simulink library "pixhawk_slib_uORB_RW"  (R2017b)
settings: Solver=ode45  StartTime=0.0  StopTime=10.0  RelTol=1e-3
undefined symbols (not defined in the file or in its folder): UNDEFINED, uORB_StuctParams
settings Model: Creator=skuznick  LastModifiedBy=uavcs
settings DataIOCC: LimitDataPoints=on  SaveFormat=Array
settings OptimizationCC: BlockReduction=off  BooleanDataType=off  LifeSpan=inf
settings DebuggingCC: SaveWithParameterizedLinksMsg=none  UnderspecifiedInitializationDetection=Classic  MergeDetectMultiDrivingBlocksExec=none  SignalResolutionControl=TryResolveAllWithWarning  AllowSymbolicDim=off  StrictBusMsg=Warning  SFUnexpectedBacktrackingDiag=warning  SFNoUnconditionalDefaultTransitionDiag=warning  SFExecutionAtInitializationDiag=none
settings HardwareCC: ProdBitPerPointer=32  ProdBitPerSizeT=32  ProdBitPerPtrDiffT=32  ProdLargestAtomicFloat=None  ProdIntDivRoundTo=Undefined  ProdEndianess=Unspecified  ProdWordSize=32  ProdHWDeviceType=32-bit Generic  TargetUnknown=on
settings ModelReferenceCC: PropagateSignalLabelsOutOfModel=off
settings CodeAppCC: StateflowObjectComments=on
settings GRTTargetCC: TargetLangStandard=C89/C90 (ANSI)  GeneratePreprocessorConditionals=Disable all
settings ConfigComp: CovMetricSettings=dw  CovHtmlReporting=on  CovSaveCumulativeToWorkspaceVar=on  CovSaveSingleToWorkspaceVar=on  CovExternalEMLEnable=off  CovSFcnEnable=off

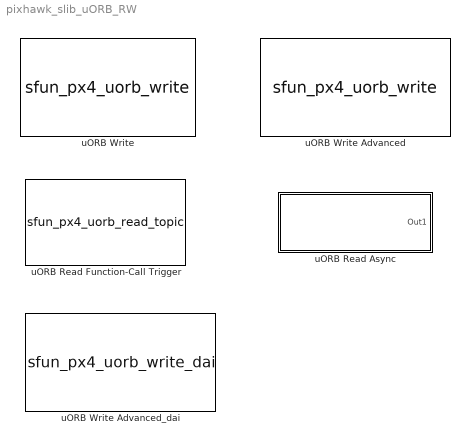
== system pixhawk_slib_uORB_RW ==
  uORB Read Async : Subsystem  mask{uORB_Topic_str=UNDEFINED, BusObjVar=Bus: actuator_armed_SL}
      mask prompts: BusObjVar "Enter Bus Object"
      mask help:
      | uORB Read Input Block
      |
      | Subscribes to a user provided named tropic structure.
      mask init:
      | ParentSubsystem = getSimulinkBlockHandle(get(gcbh,'parent'));
      | ParentConnection = [];
      | h_ParentSourceBlk = [];
      | err = 0;
      | if (ParentSubsystem~=-1)
      |     ParentConnection = get(ParentSubsystem,'PortConnectivity');
      | else
      |     set_param(gcb,'uORB_Topic_str','UNDEFINED');
      |     err = 1;
      | end
      | 
      | if ~isempty(ParentConnection)
      |     %Find which source block is the trigger
      |     for trigger_indx = 1:length(ParentConnection)
      |         if isequal(ParentConnection(trigger_indx).Type,'trigger')
      |             h_ParentSourceBlk = ParentConnection(trigger_indx).SrcBlock;
      |         end
      |     end
      | else
      |     set_param(gcb,'uORB_Topic_str','UNDEFINED');
      |     err = 1;
      | end
      | 
      | if ~isempty(h_ParentSourceBlk)
      | 
      |     Blk_Connections = get(h_ParentSourceBlk,'PortConnectivity');   
      | 
      |     while (1)
      |         Blk_Connections = get(h_ParentSourceBlk,'PortConnectivity');    
      |         if isempty(Blk_Connections(1).SrcBlock)
      |             break
      |         else    
      |             h_ParentSourceBlk =  Blk_Connections(1).SrcBlock;
      |         end
      | 
      |     end
      | 
      |     try
      |         GrabDataFrom_This_Topic = get(h_ParentSourceBlk,'uORB_Topic_str');
      |         fprintf('Function Trigger \n Topic ID: %s \n',GrabDataFrom_This_Topic);
      |         set_param(gcb,'uORB_Topic_str',GrabDataFrom_This_Topic);
      | 
      | 
      |         TopicString  = get_param(gcb,'uORB_Topic_str');
      | 
      |         p = Simulink.Mask.get(gcb);
      |         p.SelfModifiable = 'on';
      |         h = p.getDialogControl('DetectedTopicTitle');
      |         h.Prompt = ['Detected Topic: ' TopicString];
      | 
      |     catch
      |         err = 1;
      |     end
      |     
      |     else
      |         set_param(gcb,'uORB_Topic_str','UNDEFINED');
      |         err = 1;
      | end
      | 
      | if err == 1 && ~isequal(get(gcbh,'parent'),'uorb_blk_lib')
      |    % err_msg = 'Cannot place this block here. This block can only be used within a triggered subsystem driven by a uORB Trigger block';
      |     %error(err_msg);
      | end
      mask Help: eval('sharedhelp(''uORB Read Async')');
      mask DialogControl DescTextVar Prompt: This block will grab data affiliated with the uORB Topic which is driving the asynchronous subsystem this block resides in.
      mask DialogControl DescTextVar2 Prompt: The uORB Topic name will automatically be determined based on call-backs
      mask DialogControl Control3 Prompt: You will need to specify the bus object for this topic. The buttons below will help create this bus object as needed
      mask DialogControl DetectedTopicTitle Prompt: Detected Topic: 'differential_pressure'
      mask DialogControl Control6 Prompt: Refresh Topic Detection
      mask DialogControl Control6 Callback: set_param(bdroot,'SimulationCommand','Update');
      mask DialogControl BusCreate_Button Prompt: Use Bus Object from inherited Async Function Call Subsystem
      mask DialogControl BusCreate_Button Callback:
      | uORB_Topic_Name = get_param(gcb,'uORB_Topic_str');
      | % codertarget.pixhawk.blocks.Block_Callbacks.uORB.uORB_msgToBus(uORB_Topic_Name);
      | set_param(gcb,'BusObjVar',['Bus: ' uORB_Topic_Name(2:(end-1)) '_SL']);
      mask Display:
      | GrabDataFrom_This_Topic = get_param(gcb,'uORB_Topic_str');
      | fprintf('Function Trigger \n Topic ID: %s \n',GrabDataFrom_This_Topic);
  uORB Read Function-Call Trigger : S-Function  InitFcn=|  FunctionName=sfun_px4_uorb_read_topic  Parameters="Ts uORB_Topic_str  uORB_Interval AsyncOutput Fcn_call_select TaskName Poll_timeout BusObjVar"  SFunctionDeploymentMode=off  EnableBusSupport=off  SFcnStateName=uORB_fd  mask{uORB_Topic_str='actuator_armed', BusObjVar=Bus: actuator_armed_SL, uORB_Interval=4, AsyncOutput=off, Fcn_call_select=Generate Function Call Signal, TaskName='Task1', Poll_timeout=-1, Ts=-1}
      | uORB_Topic_Name = get_param(gcb,'uORB_Topic_str');
      | err = codertarget.pixhawk.blocks.Block_Callbacks.uORB.uORB_msgToBus(uORB_Topic_Name);
      | if err
      |     err_msg =[' The uORB Topic you have selected contains reference to C++ static variables.',...
      |              ' This is not supported because Embedded Coder generates',...
      |              ' C-code and therefore structs in the generated code would not be able to adapt to',...
      |              ' to this C++ data structure']
      |     error(err_msg);
      | end
      | 
      | msg_file = uORB_Topic_Name(2:(end-1));
      | msg_file=regexprep(msg_file,'_\d+$','');
      | msg_file=regexprep(msg_file,'__\w+$','');
      | msg_file=regexprep(msg_file,'#.*$','');
      | set_param(gcb,'BusObjVar',['Bus: ' msg_file '_SL'])
      | clear err;
      mask prompts: uORB_Topic_str "uORB Topic"; BusObjVar "Enter Bus Object"; uORB_Interval "uORB Interval (ms)"; AsyncOutput "Function-Call Trigger"; Fcn_call_select "Function-Call Source/Sink"; Poll_timeout "Polling Timeout (ms)  (-1 = indefinite wait, 0 = return immediately)"; Ts "Sample Time (-1 inherited)"
      mask help:
      | uORB Read Output Block
      |
      | Subscribes to user supplied topic, outputs a structure.
      mask init:
      | %Ensure timeout and uORB_interval are integer values
      | 
      | uORB_Interval = int32(uORB_Interval);
      | Poll_timeout = int32(Poll_timeout);
      settings: SFcnIsStateOwnerBlock=on
      mask Help: eval('sharedhelp(''uORB Read Function-Call Trigger')');
      mask Callback AsyncOutput: codertarget.pixhawk.blocks.Block_Callbacks.uORB.uORB_Read_Mask_UI_enable(gcbh)
      mask TypeOptions Fcn_call_select: Generate Function Call Signal | Fetch data within function-call subsystem
      mask DialogControl DescGroupVar Prompt: uORB Read and Function-Call Trigger
      mask DialogControl EntryGroupBox Prompt: This block operates in two modes:
      mask DialogControl Control5 Prompt: Mode1: Reading uORB Data
      mask DialogControl Control6 Prompt: In this mode, the block will fetch data using a uORB_CHECK( ) call and write the data to a struct. This struct is accessed as a bus object.  The buttons below allow one to create bus objects for any arbitrary uORB message provided it is specified in a .msg format. Header files are added to the generated code from: C:\px4\Firmware\src\modules\uORB\topics
      mask DialogControl Control9 Prompt: Mode2: Asynchronous Tasking
      mask DialogControl Control10 Prompt: In this mode, the block will spawn a thread which will be data-driven. When a uORB message of the specified topic arrives, the thread will advance in execution and run the contents of the affiliated function-call subsystem
      mask DialogControl msg_file_open Prompt: Open .msg file
      mask DialogControl msg_file_open Callback:
      | StrTmp = get(gcbh,'uORB_Topic_str');
      | msg_file=StrTmp(2:(end-1));
      | msg_file=regexprep(msg_file,'_\d+$','');
      | msg_file=regexprep(msg_file,'__.*$','');
      | open([codertarget.pixhawk.internal.getPX4RootDir,filesep,'Firmware' filesep 'msg' filesep msg_file '.msg' ]);
      mask DialogControl ui_open_msg_path Prompt: Select uORB Topic msg
      mask DialogControl ui_open_msg_path Callback:
      | file_path = fullfile(codertarget.pixhawk.internal.getPX4RootDir,'Firmware','msg');
      | [MsgFile_Name_ext, ~,~] = uigetfile([file_path,filesep,'*.msg']);
      | 
      | if (MsgFile_Name_ext~=0)
      |     [~, MsgFile_Name]=fileparts(MsgFile_Name_ext);
      |     set_param(gcb,'uORB_Topic_str',['''' MsgFile_Name ''''] );
      | end
      mask DialogControl BusCreate_Button Prompt: Create Bus Object
      mask DialogControl BusCreate_Button Callback:
      | uORB_Topic_Name = get_param(gcb,'uORB_Topic_str');
      | err = codertarget.pixhawk.blocks.Block_Callbacks.uORB.uORB_msgToBus(uORB_Topic_Name);
      | if err
      |     err_msg =[' The uORB Topic you have selected contains reference to C++ static variables.',...
      |              ' This is not supported because Embedded Coder generates',...
      |              ' C-code and therefore structs in the generated code would not be able to adapt to',...
      |              ' to this C++ data structure']
      |     error(err_msg);
      | end
      | msg_file = uORB_Topic_Name(2:(end-1));
      | msg_file=regexprep(msg_file,'_\d+$','');
      | msg_file=regexprep(msg_file,'__\w+$','');
      | set_param(gcb,'BusObjVar',['Bus: ' msg_file '_SL'])
      | clear err;
      mask DialogControl SubGroupBox Prompt: Function-Call Options
      mask Display:
      | Topic_name = get_param(gcb,'uORB_Topic_str');
      | AsyncOutput = get_param(gcb,'AsyncOutput');
      | 
      | Topic_name=regexprep(Topic_name,'^.*__','');
      | 
      | blk_title_str = sprintf('uORB Read Topic: \n %s',Topic_name);
      | blk_title_fcn_str =  sprintf('uORB Read - Function Trigger: \n %s',Topic_name);
      | if strcmp(AsyncOutput,'on')
      |     %Async output
      |     disp(blk_title_fcn_str);
      | else
      |     %Normal read
      |     disp(blk_title_str);
      | end
  uORB Write : S-Function  FunctionName=sfun_px4_uorb_write  Parameters="Ts,uORB_Topic_str,uORB_Struct_DT,BlockOutputCount,uORB_StuctParams, uORB_PortSizes,  uint32(0),uint32(MsgSizeOf)"  SFunctionDeploymentMode=off  EnableBusSupport=off  SFcnStateName=uorb_msg  mask{uORB_Topic_str='actuator_outputs', BlockOutputCount=2, OutputBoolean_1=on, uORB_Param_Name1='noutputs', uORB_Param_Name_DT1=uint32, VectorScalar_1=1, OutputBoolean_2=on, uORB_Param_Name2='output', uORB_Param_Name_DT2=single, VectorScalar_2=16, OutputBoolean_3=off, uORB_Param_Name3='timestamp_time', uORB_Param_Name_DT3=double, VectorScalar_3=1, OutputBoolean_4=off, uORB_Param_Name4='gyro_temp', uORB_Param_Name_DT4=single, VectorScalar_4=3, OutputBoolean_5=off, uORB_Param_Name5='vel_ned_valid', uORB_Param_Name_DT5=boolean, VectorScalar_5=1, Ts=-1, MsgSizeOf=0}
      mask prompts: uORB_Topic_str "uORB Topic"; BlockOutputCount "Number of Outputs"; OutputBoolean_1 "Input Struct param :"; VectorScalar_1 "Number of Elements"; OutputBoolean_2 "Input Struct param :"; VectorScalar_2 "Number of Elements"; OutputBoolean_3 "Input Struct param :"; VectorScalar_3 "Number of Elements"; OutputBoolean_4 "Input Struct param :"; VectorScalar_4 "Element Count"; OutputBoolean_5 "Input Struct param :"; VectorScalar_5 "Number of Elements"; Ts "Sample Time (-1 inherited)"
      mask help:
      | uORB Write Output Block
      |
      | Publishes to a user provided named tropic structure.
      mask init:
      | MaxParameters = 5;
      | 
      | uORB_DataTypes = [];
      | Visibility_Cells = get_param(gcb,'MaskVisibilities');
      | for i = 1:MaxParameters
      |     DT_Str = get_param(gcb,['uORB_Param_Name_DT' num2str(i)]);
      |     if strcmp(Visibility_Cells{5 + 4*(i-1)},'on')
      |        % EnumVal = Determine_DataType_(DT_Str);
      |             switch(DT_Str)
      |             case 'double'
      |                 EnumVal = 0;
      |             case 'single'
      |                 EnumVal = 1;
      |             case 'int8'
      |                 EnumVal = 2;
      |             case 'uint8'
      |                 EnumVal = 3;
      |             case 'int16'
      |                 EnumVal = 4;
      |             case 'uint16'
      |                 EnumVal = 5;
      |             case 'int32'
      |                 EnumVal = 6;
      |             case 'uint32'
      |                 EnumVal = 7;
      |             case 'boolean'
      |                 EnumVal = 8;
      |             end
      |     
      |         uORB_DataTypes = [uORB_DataTypes ;EnumVal];
      |     end
      | end
      | 
      | %Create array storing data type info of each output port using enum
      | %uORB_Struct_DT = uORB_DataTypes;
      | 
      | %Concantonate Parameters together
      | %[~, uORB_StuctParams] = uORB_Collect_ParamStrings(gcb,MaxParameters);
      | [ uORB_Struct_DT, uORB_PortSizes,uORB_StuctParams ] = codertarget.pixhawk.blocks.Block_Callbacks.uORB.uORB_Write_Call_Mask_Options(gcbh);
      | %Pass in parameter that will dictate if block emits function call signal or
      | %just data to be read inside function-call subsystem
      | % Fcn_Call_Or_Src = int32(strcmp(get_param(gcb,'Fcn_call_select'),'Fetch data within function-call subsystem'));
      | 
      | %Assertion Checks
      | uORB_Struct_DT = int32(uORB_Struct_DT);
      | BlockOutputCount = int32(BlockOutputCount);
      | % uORB_Interval = int32(uORB_Interval);
      | uORB_PortSizes = int32(uORB_PortSizes);
      | validateattributes(uORB_Topic_str,{'char'},{'nonempty'});
      | validateattributes(uORB_Param_Name1,{'char'},{'nonempty'});
      | validateattributes(uORB_Param_Name2,{'char'},{'nonempty'});
      | validateattributes(uORB_Param_Name3,{'char'},{'nonempty'});
      | validateattributes(uORB_Param_Name4,{'char'},{'nonempty'});
      | validateattributes(uORB_Param_Name5,{'char'},{'nonempty'});
      | 
      | 
      | MsgSizeOf = 0;
      | msg_file = uORB_Topic_str;
      | msg_file=regexprep(msg_file,'_\d+$','');
      | msg_file=regexprep(msg_file,'__.*$','');
      | path_to_msg = fullfile(codertarget.pixhawk.internal.getPX4RootDir,'Firmware','msg',[msg_file '.msg' ]);
      | [~,~,MsgSizeOf] = codertarget.pixhawk.blocks.Block_Callbacks.uORB.uORB_ParseMsgFile(path_to_msg);
      settings: SFcnIsStateOwnerBlock=on
      mask Help: eval('sharedhelp(''uORB Write'')');
      mask Callback OutputBoolean_1: [~,~,~] = codertarget.pixhawk.blocks.Block_Callbacks.uORB.uORB_Write_Call_Mask_Options(gcb);
      mask Callback OutputBoolean_2: [~,~,~] = codertarget.pixhawk.blocks.Block_Callbacks.uORB.uORB_Write_Call_Mask_Options(gcb);
      mask Callback OutputBoolean_3: [~,~,~] = codertarget.pixhawk.blocks.Block_Callbacks.uORB.uORB_Write_Call_Mask_Options(gcb);
      mask Callback OutputBoolean_4: [~,~,~] = codertarget.pixhawk.blocks.Block_Callbacks.uORB.uORB_Write_Call_Mask_Options(gcb);
      mask Callback OutputBoolean_5: [~,~,~] = codertarget.pixhawk.blocks.Block_Callbacks.uORB.uORB_Write_Call_Mask_Options(gcb);
      mask DialogControl msg_file_open Prompt: Open .msg file
      mask DialogControl msg_file_open Callback:
      | StrTmp = get(gcbh,'uORB_Topic_str');
      | msg_file = StrTmp(2:(end-1));
      | msg_file=regexprep(msg_file,'_\d+$','');
      | msg_file=regexprep(msg_file,'__.*$','');
      | open([codertarget.pixhawk.internal.getPX4RootDir,filesep,'Firmware' filesep 'msg' filesep msg_file '.msg' ]);
      mask DialogControl ui_open_msg_path Prompt: Open .msg folder
      mask DialogControl ui_open_msg_path Callback: uiopen(fullfile(codertarget.pixhawk.internal.getPX4RootDir,filesep,'Firmware',filesep,'msg',filesep,'*.msg'));
      mask DialogControl Title Prompt: uORB Parameter Names and Data Type
      mask Display:
      | %get_param(gcb,'uORB_Topic_str')
      | uORB_name=get_param(gcb,'uORB_Topic_str')
      | uORB_name=regexprep(uORB_name,'^.*__','');
      | 
      | fprintf('uORB Write \n Topic: %s ',uORB_name)
      | idx = 1;
      | 
      |     show_port = get_param(gcb,'OutputBoolean_1');
      |     if strcmp(show_port,'on') == true
      |         port_label('input', idx, get_param(gcb,'uORB_Param_Name1'));
      |         idx = idx + 1;
      |     end
      |     show_port = get_param(gcb,'OutputBoolean_2');
      |     if strcmp(show_port,'on') == true
      |         port_label('input', idx, get_param(gcb,'uORB_Param_Name2'));
      |         idx = idx + 1;
      |     end
      |     show_port = get_param(gcb,'OutputBoolean_3');
      |     if strcmp(show_port,'on') == true
      |         port_label('input', idx, get_param(gcb,'uORB_Param_Name3'));
      |         idx = idx + 1;
      |     end
      |     show_port = get_param(gcb,'OutputBoolean_4');
      |     if strcmp(show_port,'on') == true
      |         port_label('input', idx, get_param(gcb,'uORB_Param_Name4'));
      |         idx = idx + 1;
      |     end
      |     show_port = get_param(gcb,'OutputBoolean_5');
      |     if strcmp(show_port,'on') == true
      |         port_label('input', idx, get_param(gcb,'uORB_Param_Name5'));
      |         idx = idx + 1;
      |     end
  uORB Write Advanced : S-Function  FunctionName=sfun_px4_uorb_write  Parameters=Ts, uORB_Topic_str, int32(uORB_Struct_DT), int32(BlockInputCount),char(uORB_StructParams),int32(uORB_PortSizes),uint32(uORB_AdvtQueue),uint32(MsgSizeOf)  SFunctionDeploymentMode=off  EnableBusSupport=off  SFcnStateName=uorb_msg  mask{Ts=0, uORB_AdvtQueue=on, uORB_FieldEnabledArr=0  0  0  1  0  0  0  0  0  0  0, uORB_Topic_str=0, uORB_Struct_DT=[1  1  1  1  1], BlockInputCount=5, uORB_StructParams=["voltage_v","voltage_filtered_v","current_a","current_filtered_a","remaining"], uORB_PortSizes=[1  1  1  1], MsgSizeOf=0, MW_update=true}
      mask help:
      | uORB Write Output Block
      |
      | Publishes to a user provided named tropic structure.
      mask init:
      | % A structure of data can be stored in the block UserData
      | maskData = get_param(gcb,'UserData');
      | % Block Param formatted string
      | if isfield(maskData,'uORBMsg')
      |     uORB_Topic_str = maskData.uORBMsg;
      | else
      |     uORB_Topic_str = '<unformatted_placeholder_param>';
      | end
      | 
      | if isfield(maskData,'SFuncParam_DTArr')
      |     uORB_Struct_DT = maskData.SFuncParam_DTArr;
      | else
      |     uORB_Struct_DT = [1];
      | end
      | 
      | if isfield(maskData,'SFuncParam_InputCount')
      |     BlockInputCount = maskData.SFuncParam_InputCount;
      | else
      |     BlockInputCount = '["<unformatted_placeholder_param>"]';
      | end
      | 
      | % NumParams
      | if isfield(maskData,'SFuncParam_PortSizes')
      |     uORB_PortSizes =  maskData.SFuncParam_PortSizes;
      | else
      |     uORB_PortSizes = 1;
      | end
      | 
      | if isfield(maskData,'FieldEnabled')
      |     uORB_FieldEnabledArr = maskData.FieldEnabled;
      | else
      |     uORB_FieldEnabledArr = [true];
      | end
      | 
      | if isfield(maskData,'SFuncParam_TLCStr')
      |     uORB_StructParams = maskData.SFuncParam_TLCStr;
      | else
      |     uORB_StructParams = [];
      | end
      | 
      | % Sample-time
      | if isfield(maskData,'Ts') 
      |     try
      |         Ts = evalin('base',maskData.Ts);
      |     catch
      |         Ts = -1;
      |     end
      | else
      |     Ts = -1;
      | end
      | 
      | % Advt Queue
      | if isfield(maskData,'AdvtQueue') 
      |     try
      |         uORB_AdvtQueue = evalin('base',maskData.AdvtQueue);
      |     catch
      |         uORB_AdvtQueue = 0;
      |     end
      | else
      |     uORB_AdvtQueue = 0;
      | end
      | 
      | % Force parameter data type
      | Ts = double(Ts);
      | uORB_FieldEnabledArr = boolean(uORB_FieldEnabledArr);
      | uORB_Topic_str = char(uORB_Topic_str);
      | uORB_Struct_DT = int32(uORB_Struct_DT);
      | BlockInputCount = int32(BlockInputCount);
      | uORB_StructParams = char(uORB_StructParams);
      | uORB_PortSizes = int32(uORB_PortSizes);
      | uORB_AdvtQueue = uint32(uORB_AdvtQueue);
      | 
      | % Get the size of the msg struct
      | MsgSizeOf = 0;
      | msg_file = uORB_Topic_str;
      | msg_file=regexprep(msg_file,'_\d+$','');
      | msg_file=regexprep(msg_file,'__.*$','');
      | path_to_msg = fullfile(codertarget.pixhawk.internal.getPX4RootDir,'Firmware','msg',[msg_file '.msg' ]);
      | [~,~,MsgSizeOf] = codertarget.pixhawk.blocks.Block_Callbacks.uORB.uORB_ParseMsgFile(path_to_msg);
      | %debug: fprintf('Byte Value = %d \n',MsgSizeOf);
      settings: OpenFcn=codertarget.pixhawk.blocks.Block_Callbacks.uORB.ParamUpdateMaskDialog_uORB_Write(gcbh);  SFcnIsStateOwnerBlock=on
      mask Help: eval('sharedhelp(''uORB Write Advanced')');
      mask Display:
      | maskData = get_param(gcb,'UserData');
      | 
      | uORB_name=maskData.uORBMsg
      | uORB_name=regexprep(uORB_name,'^.*__','');
      | fprintf('uORB Write \n Topic: %s ',uORB_name)
      | 
      | InputStrSrc = maskData.SFuncParam_TLCStr;
      | 
      | [idx_start,idx_end] = regexp(InputStrSrc,'\"([^\"]*)\"');
      | 
      | NumOfInputs = length(idx_start);
      | 
      | for idx = 1:NumOfInputs
      |     PortName = InputStrSrc(idx_start(idx):idx_end(idx));
      |     PortName = strrep(PortName,'"','');
      |     port_label('input',idx,PortName);
      | end
  uORB Write Advanced_dai : S-Function  AncestorBlock=pixhawk_slib_uORB_RW/uORB Write Advanced  FunctionName=sfun_px4_uorb_write_dai  Parameters=Ts, uORB_Topic_str, int32(uORB_Struct_DT), int32(BlockInputCount),char(uORB_StructParams),int32(uORB_PortSizes),uint32(uORB_AdvtQueue),uint32(MsgSizeOf),uORB_Topic_str_ID  SFunctionDeploymentMode=off  EnableBusSupport=off  SFcnStateName=uorb_msg  mask{Ts=0, uORB_AdvtQueue=on, uORB_FieldEnabledArr=0  0  0  1  0  0  0  0  0  0  0, uORB_Topic_str=0, uORB_Topic_str_ID=0, uORB_Struct_DT=[1  1  1  1  1], BlockInputCount=5, uORB_StructParams=["voltage_v","voltage_filtered_v","current_a","current_filtered_a","remaining"], uORB_PortSizes=[1  1  1  1], MsgSizeOf=0, MW_update=true}
      mask help:
      | uORB Write Output Block
      |
      | Publishes to a user provided named tropic structure.
      mask init:
      | % A structure of data can be stored in the block UserData
      | maskData = get_param(gcb,'UserData');
      | % Block Param formatted string
      | if isfield(maskData,'uORBMsg')
      |     uORB_Topic_str = maskData.uORBMsg;
      | else
      |     uORB_Topic_str = '<unformatted_placeholder_param>';
      | end
      | 
      | if isfield(maskData,'uORBMsgID')  % edited by Daidai
      |     uORB_Topic_str_ID = maskData.uORBMsgID;  % edited by Daidai
      | else  % edited by Daidai
      |     uORB_Topic_str_ID = uORB_Topic_str;  % edited by Daidai
      | end  % edited by Daidai
      | 
      | if isfield(maskData,'SFuncParam_DTArr')
      |     uORB_Struct_DT = maskData.SFuncParam_DTArr;
      | else
      |     uORB_Struct_DT = [1];
      | end
      | 
      | if isfield(maskData,'SFuncParam_InputCount')
      |     BlockInputCount = maskData.SFuncParam_InputCount;
      | else
      |     BlockInputCount = '["<unformatted_placeholder_param>"]';
      | end
      | 
      | % NumParams
      | if isfield(maskData,'SFuncParam_PortSizes')
      |     uORB_PortSizes =  maskData.SFuncParam_PortSizes;
      | else
      |     uORB_PortSizes = 1;
      | end
      | 
      | if isfield(maskData,'FieldEnabled')
      |     uORB_FieldEnabledArr = maskData.FieldEnabled;
      | else
      |     uORB_FieldEnabledArr = [true];
      | end
      | 
      | if isfield(maskData,'SFuncParam_TLCStr')
      |     uORB_StructParams = maskData.SFuncParam_TLCStr;
      | else
      |     uORB_StructParams = [];
      | end
      | 
      | % Sample-time
      | if isfield(maskData,'Ts') 
      |     try
      |         Ts = evalin('base',maskData.Ts);
      |     catch
      |         Ts = -1;
      |     end
      | else
      |     Ts = -1;
      | end
      | 
      | % Advt Queue
      | if isfield(maskData,'AdvtQueue') 
      |     try
      |         uORB_AdvtQueue = evalin('base',maskData.AdvtQueue);
      |     catch
      |         uORB_AdvtQueue = 0;
      |     end
      | else
      |     uORB_AdvtQueue = 0;
      | end
      | 
      | % Force parameter data type
      | Ts = double(Ts);
      | uORB_FieldEnabledArr = boolean(uORB_FieldEnabledArr);
      | uORB_Topic_str = char(uORB_Topic_str);
      | uORB_Topic_str_ID = char(uORB_Topic_str_ID);  %edited by Daidai
      | uORB_Struct_DT = int32(uORB_Struct_DT);
      | BlockInputCount = int32(BlockInputCount);
      | uORB_StructParams = char(uORB_StructParams);
      | uORB_PortSizes = int32(uORB_PortSizes);
      | uORB_AdvtQueue = uint32(uORB_AdvtQueue);
      | 
      | % Get the size of the msg struct
      | MsgSizeOf = 0;
      | path_to_msg = fullfile(codertarget.pixhawk.internal.getPX4RootDir,'Firmware','msg',[uORB_Topic_str '.msg' ]);
      | [~,~,MsgSizeOf] = codertarget.pixhawk.blocks.Block_Callbacks.uORB.uORB_ParseMsgFile(path_to_msg);
      | %debug: fprintf('Byte Value = %d \n',MsgSizeOf);
      settings: OpenFcn=codertarget.pixhawk.blocks.Block_Callbacks.uORB.ParamUpdateMaskDialog_uORB_Write_dai(gcbh);  SFcnIsStateOwnerBlock=on
      mask Help: eval('sharedhelp(''uORB Write Advanced_dai')');
      mask Display:
      | maskData = get_param(gcb,'UserData');
      | 
      | if isfield(maskData,'uORBMsgID')  % edited by Daidai
      |     uORB_strID = maskData.uORBMsgID;  % edited by Daidai
      | else  % edited by Daidai
      |     uORB_strID = maskData.uORBMsg;  % edited by Daidai
      | end  % edited by Daidai
      | 
      | fprintf('uORB Write_dai \n Topic: %s ',uORB_strID)
      | 
      | InputStrSrc = maskData.SFuncParam_TLCStr;
      | 
      | [idx_start,idx_end] = regexp(InputStrSrc,'\"([^\"]*)\"');
      | 
      | NumOfInputs = length(idx_start);
      | 
      | for idx = 1:NumOfInputs
      |     PortName = InputStrSrc(idx_start(idx):idx_end(idx));
      |     PortName = strrep(PortName,'"','');
      |     port_label('input',idx,PortName);
      | end

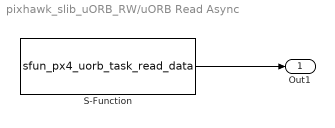
== system pixhawk_slib_uORB_RW/uORB Read Async ==
  S-Function : S-Function  FunctionName=sfun_px4_uorb_task_read_data  Parameters=uORB_Topic_str,BusObjVar  SFunctionDeploymentMode=off  EnableBusSupport=off
  Out1 : Outport
  wires:
  S-Function/1 -> Out1/1
